simulink library "SetDsm"  (R2022b)
settings: Solver=VariableStepAuto  StartTime=0.0  StopTime=10.0  RelTol=1e-3
libraries: simulink x1
settings Model: Creator=kl13806  LastModifiedBy=kl13806

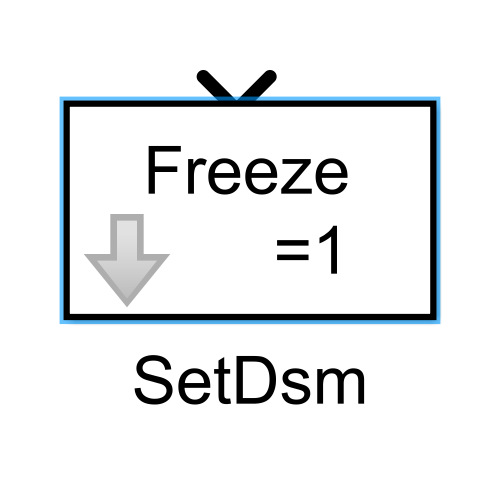
[thumbnail: Simulink's stored preview of the top-level diagram]
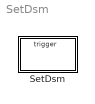
== system SetDsm ==
  SetDsm : Subsystem  mask(Talaria Set DSM){DataStoreName=Freeze, Value=uint32(1), SampleTime=-1}
      mask prompts: DataStoreName "Simulink:blkprm_prompts:DstoreMemDstoreName"; Value "Simulink:blkprm_prompts:ConstConstValue"; SampleTime "Sample time to lock:"
      mask help: SetDsm only contains a function trigger and a Data Store Write but with a twist: its Code Generation settings specify to create a function. This critical detail enables multiple DSM writes to happen within a single frame such as when subversive asynchronous tasks wish to signal the periodic full rate tasks to stay away from ramping variables. Otherwise code optimization is very likely to eliminate all but the final write to the DSM.
      mask Help:
      | Provide the name of the Data Store Memory (the DSM name, not the block name) and a value to write into the DSM.
      | If provided (i.e. greater-than 0) then the specified rate will be located in the model's call rates. Otherwise, the base rate is assumed. The locking directives in generated code reference the relevant task ID as a functional argument.
      mask TypeOptions DataStoreName:
      | DsmWrite/Data Store
      | Write/DataStoreName
      mask TypeOptions Value: DsmWrite/Constant/Value
      mask DialogControl DataStoreName Prompt: Data store name:
      mask DialogControl Value Prompt: Constant value:
      mask Display: fprintf('%s\n       =%d',DataStoreName,Value);

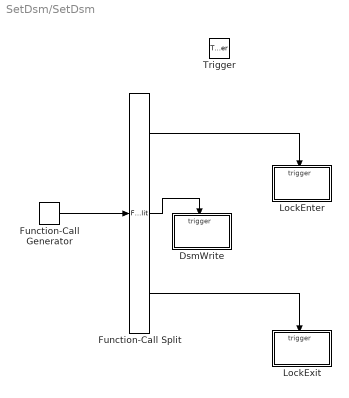
== system SetDsm/SetDsm ==
  Trigger : TriggerPort  TriggerType=function-call  FunctionName=TheBigOne  VariantControl=(inherit)  PortDimensions=1
  DsmWrite : Subsystem
  Function-Call Generator : simulink/Ports & Subsystems/Function-Call Generator  sample_time=-1  numberOfIterations=1  DisallowWideOutput=off
  Function-Call Split : FunctionCallSplit  IconShape=distinctive  NumOutputPorts=3  OutputPortLayout=default
  LockEnter : Subsystem  TreatAsAtomicUnit=on
  LockExit : Subsystem  TreatAsAtomicUnit=on
  wires:
  Function-Call Split/1 -> LockEnter/Trigger
  Function-Call Split/2 -> DsmWrite/Trigger
  Function-Call Split/3 -> LockExit/Trigger
  Function-Call Generator/1 -> Function-Call Split/1

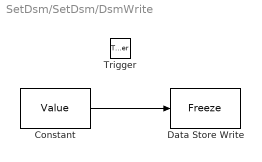
== system SetDsm/SetDsm/DsmWrite ==
  Trigger : TriggerPort  TriggerType=function-call  FunctionName=TheBigOne  VariantControl=(inherit)  PortDimensions=1
  Constant : Constant  Value=Value
  Data Store Write : DataStoreWrite  DataStoreName=Freeze  IndexOptions=Index vector (dialog)  Indices=1  OutputSizes=1
  wires:
  Constant/1 -> Data Store Write/1

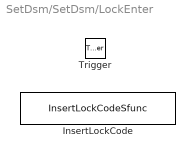
== system SetDsm/SetDsm/LockEnter ==
  Trigger : TriggerPort  TriggerType=function-call  VariantControl=(inherit)
  InsertLockCode : M-S-Function  FunctionName=InsertLockCodeSfunc  Parameters=1,SampleTime

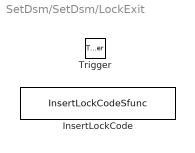
== system SetDsm/SetDsm/LockExit ==
  Trigger : TriggerPort  TriggerType=function-call  VariantControl=(inherit)
  InsertLockCode : M-S-Function  FunctionName=InsertLockCodeSfunc  Parameters=0,SampleTime
